simulink subsystem "Simple_spring_and_damper"  (R2025b)
settings: Solver=VariableStepAuto  StartTime=0.0  StopTime=10.0  RelTol=1e-3
undefined symbols (not defined in the file): cz, kz
settings Model: Creator=The MathWorks, Inc.  LastModifiedBy=The MathWorks, Inc.
settings RTWCC: GPUComputeCapability=3.5

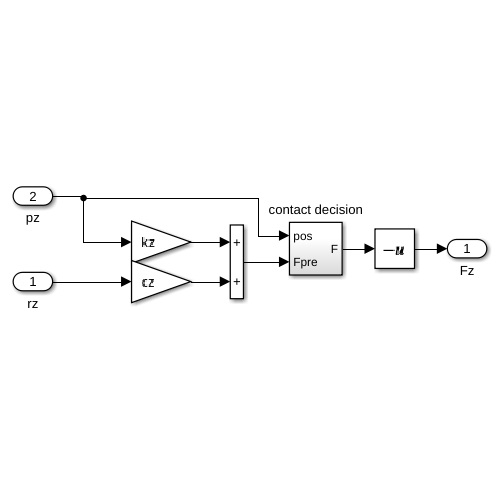
[thumbnail: Simulink's stored preview of the top-level diagram]
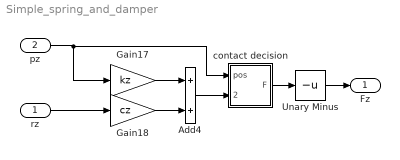
== system Simple_spring_and_damper ==
  rz : Inport
  pz : Inport  Port=2
  Add4 : Sum
  Gain17 : Gain  Gain=kz
  Gain18 : Gain  Gain=cz
  Unary Minus : UnaryMinus
  contact decision : Subsystem
  Fz : Outport
  wires:
  Unary Minus/1 -> Fz/1
  rz/1 -> Gain18/1
  Gain18/1 -> Add4/2
  contact decision/1(F) -> Unary Minus/1
  Add4/1 -> contact decision/2(Fpre)
  Gain17/1 -> Add4/1
  pz/1 -> Gain17/1, contact decision/1(pos)

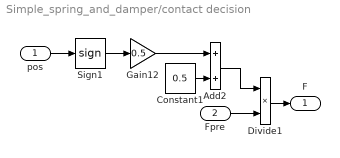
== system Simple_spring_and_damper/contact decision ==
  pos : Inport
  Fpre : Inport  Port=2
  Add2 : Sum
  Constant1 : Constant  Value=0.5
  Divide1 : Product  Inputs=**
  Gain12 : Gain  Gain=0.5
  Sign1 : Signum  ZeroCross=off
  F : Outport  VectorParamsAs1DForOutWhenUnconnected=off
  wires:
  Gain12/1 -> Add2/1
  pos/1 -> Sign1/1
  Constant1/1 -> Add2/2
  Sign1/1 -> Gain12/1
  Add2/1 -> Divide1/1
  Fpre/1 -> Divide1/2
  Divide1/1 -> F/1
